simulink library "dsparch4"  (Simulink 6.0)
settings: Solver=ode45  SolverMode=SingleTasking  StartTime=0.0  StopTime=10.0  RelTol=1e-3
values from neighbouring files (symbols this model uses):
  a = []    [dspfdes.m]    (also in dsprprim.m = a-Mi)
  b = []    [dspfdes.m]    (also in dsprprim.m = b+Li)
  c = []    [dspfdes.m]    (also in liblinks.m = cell2struct(v,f,1); sbufscop.m = 'auto')
  d = []    [dspfdes.m]    (also in dsprprim.m = ['x[' num2str(Mi) 'n/' num2str(Li) ']']; resave_mdl.m = dir('*.mdl'); sbufscop.m = abs(magMax-magMin); sdspfscope.m = get(block_data.hframenum(2),'userdata'))
  H = reshape(H,Li,Mi*Ni)    [dsprprim.m]
  N = size(cmap,1)    [sdspmview.m]
undefined symbols (not defined in the file or in its folder): bitrevorder, D, dspblkfdatool, L, M
libraries: dspmtrx3 x7, dspsigattribs x4, dspxfrm3 x4, dspbuff3 x4, dspsigops x2, dsparch4 x1, simulink x1
settings Model: Creator=hshivaku  LastModifiedBy=hshivaku  ExtModeAutoUpdateStatusClock=off  ProdHWDeviceType=Specified
settings DataIOCC: SignalLoggingName=logsOut
settings OptimizationCC: BooleanDataType=off
settings DebuggingCC: CheckExecutionContextPreStartOutputMsg=on  CheckExecutionContextRuntimeOutputMsg=on  SolverPrmCheckMsg=none
settings HardwareCC: ProdHWDeviceType=Specified  TargetUnknown=on
settings ModelReferenceCC: UpdateModelReferenceTargets=IfOutOfDate
settings SFSimCC: SFSimApplyToAllLibs=on  SFSimBuildMode=Incremental

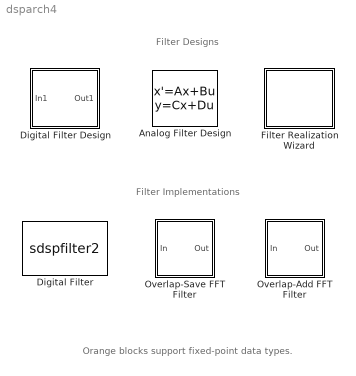
== system dsparch4 ==
  note: Filter Designs
  note: Filter Implementations
  note: Orange blocks support fixed-point data types.
  Analog Filter Design : StateSpace  A=a  B=b  C=c  D=d  mask(Analog Filter Design){method=Butterworth, filttype=Lowpass, N=8, Wlo=30, Whi=80, Rp=2, Rs=40}
      mask prompts: method "Design method:"; filttype "Filter type:"; N "Filter order:"; Wlo "Passband edge frequency (rads/sec):"; Whi "(unused)"; Rp "Passband ripple in dB:"; Rs "Stopband attenuation in dB:"
      mask help: Design one of several standard analog filters, implemented in state-space form.
      mask init:
      | [a,b,c,d,h,w,str]=dspblkanalog('design', method,filttype,N,Wlo,Whi,Rp,Rs);
      mask Help: web(dspbhelp);
      mask StyleString: popup(Butterworth|Chebyshev I|Chebyshev II|Elliptic|Bessel),popup(Lowpass|Highpass|Bandpass|Bandstop),edit,edit,edit,edit,edit
      mask CallbackString: dspblkanalog|dspblkanalog|||||
      mask Display: plot(w,h); text(.05,.9,str);
  Digital Filter Design : Subsystem  StartFcn=dspblkfdatool('StartFcn');  TreatAsAtomicUnit=on  PropExecContextAcrossSSBoundary=on
      mask init:
      | h = dspblkfdatool('initializationCommands');
      settings: ModelCloseFcn=dspblkfdatool('ModelCloseFcn');  NameChangeFcn=dspblkfdatool('NameChange');  OpenFcn=dspblkfdatool('OpenFcn');  CloseFcn=dspblkfdatool('CloseFcn');
      mask Display:
      | plot(h);
      | text(.05,.9,'FDATool')
  Digital Filter : S-Function  DialogController=dspDDGCreate  DialogControllerArgs=DataTag2  FunctionName=sdspfilter2  Parameters=a.CoeffsFromMask, a.FilterType, a.FilterStruct, a.FilterPerSample, a.a0CoeffIsUnity, a.Coeff1, a.Coeff2, a.sosCoeffs, a.scaleValues, a.IC, secondCoeffFracLength, scaleValueFracLength, tapSumMode, tapSumWordLength, tapSumFracLength, stageIOMode, stageIOWordLength, stageInFracLength, stageOutFracLength, dtInfo.firstCoeffMode, dtInfo.firstCoeffWordLength, dtInfo.firstCoeffFracLength, dtInfo.prodOutputMode, dtInfo.prodOutputWordLength, dtInfo.prodOutputFracLength, dtInfo.accumMode, dtInfo.accumWordLength, dtInfo.accumFracLength, dtInfo.memoryMode, dtInfo.memoryWordLength, dtInfo.memoryFracLength, dtInfo.outputMode, dtInfo.outputWordLength, dtInfo.outputFracLength, dtInfo.roundingMode, dtInfo.overflowMode  mask(Digital Filter){TypePopup=IIR (poles & zeros), IIRFiltStruct=Direct form II transposed, AllPoleFiltStruct=Direct form, FIRFiltStruct=Direct form, CoeffSource=Specify via dialog, NumCoeffs=[1 2], DenCoeffs=[1 0.1], BiQuadCoeffs=[1 0.3 0.4 1 0.1 0.2], LatticeCoeffs=[0.2 0.4], denIgnore=on, FiltPerSampPopup=One filter per frame, IC=0, ICnum=0, ICden=0, additionalParams=off, allowOverrides=on, showCoeff=off, firstCoeffMode=Same word length as input, firstCoeffWordLength=16, firstCoeffFracLength=15, secondCoeffMode=Same as numerator, secondCoeffWordLength=16, secondCoeffFracLength=15, thirdCoeffMode=Same as input, thirdCoeffWordLength=16, thirdCoeffFracLength=15, showOut=off, outputMode=Same as accumulator, outputWordLength=16, outputFracLength=15, showAcc=off, accumMode=Same as product output, accumWordLength=32, accumFracLength=30, showMpy=off, prodOutputMode=Same as input, prodOutputWordLength=32, prodOutputFracLength=30, showMem=off, memoryMode=Same as accumulator, memoryWordLength=16, memoryFracLength=15, roundingMode=Floor, overflowMode=off, ScaleValues=1, scaleValueFracLength=14, tapSumMode=Same as input, tapSumWordLength=32, tapSumFracLength=30, stageIOMode=Same as input, stageIOWordLength=16, stageInFracLength=15, stageOutFracLength=15, LockScale=off}
      mask prompts: TypePopup "Transfer function type:"; IIRFiltStruct "Filter structure:"; AllPoleFiltStruct "Filter structure:"; FIRFiltStruct "Filter structure:"; CoeffSource "Coefficient source:"; NumCoeffs "Numerator coefficients:"; DenCoeffs "Denominator coefficients:"; BiQuadCoeffs "SOS matrix (Mx6):"; LatticeCoeffs "Reflection coefficients:"; denIgnore "First denominator coefficient = 1, remove 1/a0 term in the structure"; FiltPerSampPopup "Coefficient update rate:"; IC "Initial conditions:"; ICnum "Initial conditions on zeros side:"; ICden "Initial conditions on poles side:"; additionalParams "------- Show additional parameters --------"; allowOverrides "Allow overrides from DSP Fixed-Point Attributes blocks"; showCoeff "------- Show coefficient fixed-point attributes --------"; firstCoeffMode "Numerator coefficient attributes:"; firstCoeffWordLength "Numerator coefficient word length:"; firstCoeffFracLength "Numerator coefficient fraction length:"; secondCoeffMode "Denominator coefficient attributes:"; secondCoeffWordLength "Denominator coefficient word length:"; secondCoeffFracLength "Denominator coefficient fraction length:"; thirdCoeffMode "Denominator coefficient attributes:"; thirdCoeffWordLength "Denominator coefficient word length:"; thirdCoeffFracLength "Denominator coefficient fraction length:"; showOut "------- Show output fixed-point attributes --------"; outputMode "Output attributes:"; outputWordLength "Output word length:"; outputFracLength "Output fraction length:"; showAcc "------- Show accumulator fixed-point attributes --------"; accumMode "Accumulator attributes:"; accumWordLength "Accumulator word length:"; accumFracLength "Accumulator fraction length:"; showMpy "------- Show product output fixed-point attributes --------"; prodOutputMode "Product output attributes:"; prodOutputWordLength "Product output word length:"; prodOutputFracLength "Product output fraction length:"; showMem "------- Show state memory fixed-point attributes --------"; memoryMode "State memory attributes:"; memoryWordLength "State memory word length:"; memoryFracLength "State memory fraction length:"; roundingMode "Round integer calculations toward:"; overflowMode "Saturate on integer overflow"; ScaleValues "Scale values:"; scaleValueFracLength "Scale value fraction length:"; tapSumMode "Tap sum attributes:"; tapSumWordLength "Tap sum word length:"; tapSumFracLength "Tap sum fraction length:"; stageIOMode "Stage IO attributes:"; stageIOWordLength "Stage IO word length:"; stageInFracLength "Stage input fraction length:"; stageOutFracLength "Stage output fraction length:"; LockScale "Lock scaling"
      mask help:
      | Independently filter each channel of the input over time using a specified digital filter implementation.  Filter coefficients can be specified using either tunable mask dialog parameters or separate input ports (useful for time-varying coefficients).
      |
      | Time-varying coefficients are supported at one of two possible rates of coefficient update in frame-based processing.  The coefficients can update at a rate of one filter per frame (i.e. they stay constant for the duration of an input frame and change for the next frame).  Or, the coefficients can update at a rate of one filter per sample (i.e. they change with every sample in the input frame).
      mask init:
      | s           = dspblkfilter('icon');
      | [a, dtInfo] = dspblkfilter('init');
      settings: CopyFcn=dspfixptcopycallback
      mask Help: web(dspbhelp);
      mask StyleString: popup(IIR (poles & zeros)|IIR (all poles)|FIR (all zeros)),popup(Direct form I|Direct form I transposed|Direct form II|Direct form II transposed|Biquad direct form I (SOS)|Biquad direct form I transposed (SOS)|Biquad direct form II (SOS)|Biquad direct form II transposed (SOS)),popup(Direct form|Direct form transposed|Lattice AR),popup(Direct form|Direct form symmetric|Direct form antisymmetric|Direct form transposed|Lattice MA),popup(Specify via dialog|Input port(s)),edit,edit,edit,edit,checkbox,popup(One filter per frame|One filter per sample),edit,edit,edit,checkbox,checkbox,checkbox,popup(Same word length as input|Specify word length|Binary point scaling|Slope and bias scaling|Same as input|User-defined),edit,edit,popup(Same as numerator|Same word length as numerator|Same word length as input|Binary point scaling|Slope and bias scaling|Same as input|User-defined),edit,edit,popup(Same word length as input|Binary point scaling|Slope and bias scaling|Same as input|User-defined),edit,edit,checkbox,popup(Same as input|Same as accumulator|Binary point scaling|Slope and bias scaling|User-defined),edit,edit,checkbox,popup(Same as input|Same as product output|Binary point scaling|Slope and bias scaling|User-defined),edit,edit,checkbox,popup(Same as input|Binary point scaling|Slope and bias scaling|User-defined),edit,edit,checkbox,popup(Same as input|Same as accumulator|Binary point scaling|Slope and bias scaling|User-defined),edit,edit,popup(Floor|Nearest),checkbox,edit,edit,popup(Same as input|Binary point scaling|Slope and bias scaling),edit,edit,popup(Same as input|Binary point scaling|Slope and bias scaling),edit,edit,edit,checkbox
      mask Display:
      | text(0.5,0.85,s.icon,'horiz','center');
      | plot(s.x, s.y);
      | port_label('input',s.i1,s.s1);
      | port_label('input',s.i2,s.s2);
      | port_label('input',1,s.in);
      | port_label('output',1,s.out);
  Filter Realization Wizard : Subsystem  PropExecContextAcrossSSBoundary=on  mask(Filter Realization Wizard){}
      mask help: Automatically construct filter realizations with specific architectures, using sum, gain, and delay blocks.
      mask init:
      | xw=[NaN 0.8 0.8 NaN 0.687 0.743 NaN 0.64 0.72 NaN 0.710 0.743 NaN 0.8 0.8 NaN 0.913 0.857 NaN 0.96 0.88 NaN 0.808 0.792 0.961 0.978 0.808 NaN 0.825 0.808 NaN 0.961 0.944];
      | yw=[NaN 0.64 0.72 NaN 0.687 0.743 NaN 0.8 0.8 NaN 0.890 0.857 NaN 0.96 0.88 NaN 0.913 0.857 NaN 0.8 0.8 NaN 0.808 0.792 0.622 0.639 0.808 NaN 0.792 0.775 NaN 0.656 0.639];
      | 
      | xl = [.1 .7 NaN .3 .3 NaN .7 .7 NaN .3 .3 NaN .7 .7 NaN .3 .9];
      | yl = [.8 .8 NaN .8 .6 NaN .8 .6 NaN .4 .2 NaN .4 .13 NaN .2 .2];
      | xz = [.46 .54 .46 NaN .54 .59 .54 .59 NaN .61 .64 NaN .67 .67];
      | yz = [.84 .8  .76 NaN .92 .92 .86 .86 NaN .93 .93 NaN .97 .89];
      | xg = [.21 .39 .3 .21 NaN .61 .79 .7 .61];
      | yg = [.6  .6  .4 .6  NaN .6  .6  .4 .6];
      | t=(0:12)/12*2*pi;
      | xs = .07*cos(t)+.7;
      | ys = .07*sin(t)+.2;
      settings: CopyFcn=dspfixptcopycallback  OpenFcn=dspfwiz
      mask Help: web(dspbhelp);
      mask Display:
      | text(.05, .9, 'FDATool');
      | plot([[xl NaN xz NaN xg NaN xs NaN]*.9-.075 xw],
      | [[yl NaN yz NaN yg NaN ys NaN]*.9-.1 yw]);
  Overlap-Add FFT Filter : Subsystem  PropExecContextAcrossSSBoundary=on  mask(Overlap-Add FFT Filter){Nfft=64, h=fir1(20,0.2), output_complexity=Real}
      mask prompts: Nfft "FFT size:"; h "FIR coefficients:"; output_complexity "Output:"
      mask help:
      | FFT based filtering using the overlap-add algorithm. Set 'Output' to 'Complex' if either the input signal or the filter coefficients are complex.
      |
      | 'FFT Size' must equal or exceed the number of filter coefficients.  Smaller FFT sizes lead to less latency but also less computational efficiency, decreasing the benefits of frequency domain processing.
      mask init:
      | [N,H,M,L] = dspblkolapfilt('init',double(Nfft),h);
      mask Help: web(dspbhelp);
      mask StyleString: edit,edit,popup(Real|Complex)
      mask Display:
      | disp('Overlap\nAdd');
      | ... plot(log10(abs(H(1:(N/2)))))
  Overlap-Save FFT Filter : Subsystem  PropExecContextAcrossSSBoundary=on  mask(Overlap-Save FFT Filter){nfft_in=64, h=fir1(20,0.2), output_complexity=Real}
      mask prompts: nfft_in "FFT size:"; h "FIR coefficients:"; output_complexity "Output:"
      mask help:
      | FFT based filtering using the overlap-save algorithm.  Set 'Output' to 'Complex' if either the input signal or the filter coefficients are complex.
      |
      | 'FFT Size' must equal or exceed the number of filter coefficients.  Smaller FFT sizes lead to less latency but also less computational efficiency, decreasing the benefits of frequency domain processing.
      mask init:
      | [N,H,M] = dspblkolapfilt('init',double(nfft_in),h);
      mask Help: web(dspbhelp);
      mask StyleString: edit,edit,popup(Real|Complex)
      mask Display:
      | disp('Overlap\nSave');
      | ... plot(log10(abs(H(1:(nfft/2)))))

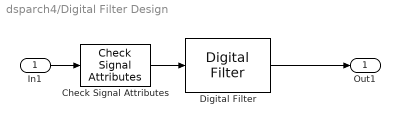
== system dsparch4/Digital Filter Design ==
  In1 : Inport  LatchInput=off
  Check Signal Attributes : dspsigattribs/Check Signal Attributes  SigAttribCheckMethod=Does not match attributes exactly  Complexity=Ignore  Frame=Ignore  DimsCheckMethod=Ignore  Dimensions=1-D  DatatypeCheckMethod=Is...  DatatypeGeneral=Floating-point  DtypeFloatSpecific=Any floating-point  DtypeFixedSpecific=Any fixed-point  DtypeIntSpecific=Any integer  SampleMode=Ignore
  Digital Filter : dsparch4/Digital Filter  DialogController=dspDDGCreate  DialogControllerArgs=DataTag1  TypePopup=FIR (all zeros)  IIRFiltStruct=Direct form II transposed  AllPoleFiltStruct=Direct form  FIRFiltStruct=Direct form  CoeffSource=Specify via dialog  NumCoeffs=[-0.00210513308421233 -0.0108086929126824 -0.0274040066202062 -0.0409457925088376 -0.0265637803556961 0.0373657306444183 0.143461670470426 0.246522720033777 0.289577286549258 0.246522720033777 0.143461670470426 0.0373657306444183 -0.0265637803556961 -0.0409457925088376 -0.0274040066202062 -0.0108086929126824 -0.00210513308421233]  DenCoeffs=[1 0.1]  BiQuadCoeffs=[1 0.3 0.4 1 0.1 0.2]  LatticeCoeffs=[0.2 0.4]  denIgnore=on  FiltPerSampPopup=One filter per frame  IC=0  ICnum=0  ICden=0  roundingMode=Floor  overflowMode=off  ScaleValues=1  scaleValueFracLength=14  stageInFracLength=15  stageOutFracLength=15
  Out1 : Outport
  wires:
  In1/1 -> Check Signal Attributes/1
  Digital Filter/1 -> Out1/1
  Check Signal Attributes/1 -> Digital Filter/1

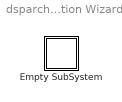
== system dsparch4/Filter Realization Wizard ==
  Empty SubSystem : Subsystem  PropExecContextAcrossSSBoundary=on

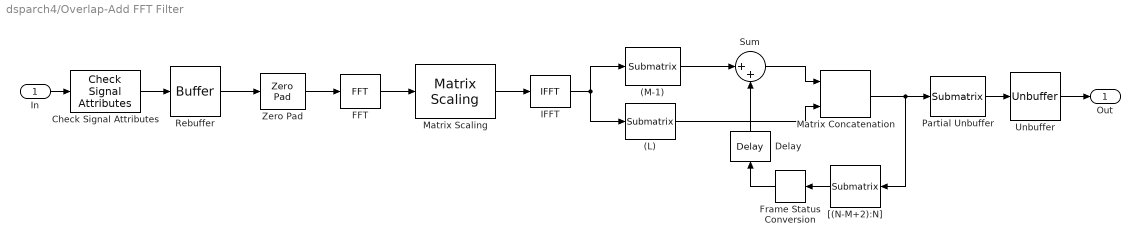
== system dsparch4/Overlap-Add FFT Filter ==
  In : Inport  LatchInput=off
  (L) : dspmtrx3/Submatrix  RowSpan=Range of rows  RowStartMode=Offset from last  RowStartIndex=L-1  RowEndMode=Last  RowEndIndex=1  ColSpan=All columns  ColStartMode=First  ColStartIndex=1  ColEndMode=Last  ColEndIndex=1
  (M-1) : dspmtrx3/Submatrix  RowSpan=Range of rows  RowStartMode=First  RowStartIndex=M-1  RowEndMode=Index  RowEndIndex=M-1  ColSpan=All columns  ColStartMode=First  ColStartIndex=1  ColEndMode=Last  ColEndIndex=1
  Check Signal Attributes : dspsigattribs/Check Signal Attributes  SigAttribCheckMethod=Does not match attributes exactly  Complexity=Ignore  Frame=Ignore  DimsCheckMethod=Ignore  Dimensions=1-D  DatatypeCheckMethod=Is...  DatatypeGeneral=Floating-point  DtypeFloatSpecific=Any floating-point  DtypeFixedSpecific=Any fixed-point  DtypeIntSpecific=Any integer  SampleMode=Ignore
  Delay : dspsigops/Delay  Orientation=up  dly_unit=Samples  delay=1  ic_detail=off  dif_ic_for_ch=off  dif_ic_for_dly=off  ic=0  reset_popup=None
  FFT : dspxfrm3/FFT  CompMethod=Table lookup  TableOpt=Speed  BitRevOrder=on  SkipNorm=on  roundingMode=Floor  overflowMode=off
      settings: allowOverrides=off
  Frame Status Conversion : dspsigattribs/Frame Status Conversion  Orientation=left  growRefPort=off  outframe=Sample-based
  IFFT : dspxfrm3/IFFT  DialogController=dspDDGCreate  DialogControllerArgs=DataTag3  CompMethod=Table lookup  TableOpt=Speed  BitRevOrder=on  cs_in=on  SkipNorm=off  mode=Real  roundingMode=Floor  overflowMode=off
      settings: allowOverrides=off
  Matrix Concatenation : simulink/Math Operations/Matrix Concatenation  numInports=2  catMethod=Vertical
  Matrix Scaling : dspmtrx3/Matrix Scaling  mode=Scale rows (D*A)  D_Source=Dialog parameter  D_VectFromMask=bitrevorder(H(:))  roundingMode=Floor  overflowMode=off
      settings: allowOverrides=off
  Partial Unbuffer : dspmtrx3/Submatrix  RowSpan=Range of rows  RowStartMode=First  RowStartIndex=M  RowEndMode=Index  RowEndIndex=L  ColSpan=All columns  ColStartMode=First  ColStartIndex=1  ColEndMode=Last  ColEndIndex=1
  Rebuffer : dspbuff3/Buffer  N=L  V=0  ic=0
  Sum : Sum  Inputs=|++  InputSameDT=on
  Unbuffer : dspbuff3/Unbuffer  ic=0
  Zero Pad : dspsigops/Zero Pad  padSigAt=End  zpadAlong=Columns  padNumOutRowsSpecMethod=User-specified  numOutRows=N  padNumOutColsSpecMethod=User-specified  numOutCols=1  trunc_flag=None
  "[(N-M+2):N]" : dspmtrx3/Submatrix  Orientation=left  RowSpan=Range of rows  RowStartMode=Index  RowStartIndex=(N-M+2)  RowEndMode=Last  RowEndIndex=N  ColSpan=All columns  ColStartMode=First  ColStartIndex=1  ColEndMode=Last  ColEndIndex=1
  Out : Outport  InitialOutput=0
  wires:
  Partial Unbuffer/1 -> Unbuffer/1
  Sum/1 -> Matrix Concatenation/1
  (M-1)/1 -> Sum/1
  Delay/1 -> Sum/2
  (L)/1 -> Matrix Concatenation/2
  "[(N-M+2):N]"/1 -> Frame Status Conversion/1
  Matrix Concatenation/1 -> Partial Unbuffer/1, "[(N-M+2):N]"/1
  Unbuffer/1 -> Out/1
  Matrix Scaling/1 -> IFFT/1
  IFFT/1 -> (L)/1, (M-1)/1
  Zero Pad/1 -> FFT/1
  Rebuffer/1 -> Zero Pad/1
  FFT/1 -> Matrix Scaling/1
  In/1 -> Check Signal Attributes/1
  Frame Status Conversion/1 -> Delay/1
  Check Signal Attributes/1 -> Rebuffer/1

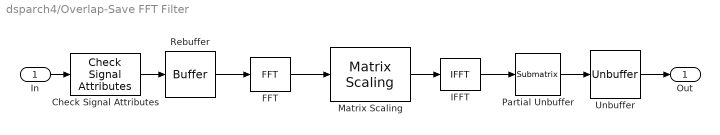
== system dsparch4/Overlap-Save FFT Filter ==
  In : Inport  LatchInput=off
  Check Signal Attributes : dspsigattribs/Check Signal Attributes  SigAttribCheckMethod=Does not match attributes exactly  Complexity=Ignore  Frame=Ignore  DimsCheckMethod=Ignore  Dimensions=1-D  DatatypeCheckMethod=Is...  DatatypeGeneral=Floating-point  DtypeFloatSpecific=Any floating-point  DtypeFixedSpecific=Any fixed-point  DtypeIntSpecific=Any integer  SampleMode=Ignore
  FFT : dspxfrm3/FFT  CompMethod=Table lookup  TableOpt=Speed  BitRevOrder=on  SkipNorm=on  roundingMode=Floor  overflowMode=off
      settings: allowOverrides=off
  IFFT : dspxfrm3/IFFT  DialogController=dspDDGCreate  DialogControllerArgs=DataTag4  CompMethod=Table lookup  TableOpt=Speed  BitRevOrder=on  cs_in=on  SkipNorm=off  mode=Real  roundingMode=Floor  overflowMode=off
      settings: allowOverrides=off
  Matrix Scaling : dspmtrx3/Matrix Scaling  mode=Scale rows (D*A)  D_Source=Dialog parameter  D_VectFromMask=bitrevorder(H(:))  roundingMode=Floor  overflowMode=off
      settings: allowOverrides=off
  Partial Unbuffer : dspmtrx3/Submatrix  RowSpan=Range of rows  RowStartMode=Index  RowStartIndex=M  RowEndMode=Last  RowEndIndex=1  ColSpan=All columns  ColStartMode=First  ColStartIndex=1  ColEndMode=Last  ColEndIndex=1
  Rebuffer : dspbuff3/Buffer  N=N  V=M-1  ic=0
  Unbuffer : dspbuff3/Unbuffer  ic=0
  Out : Outport  InitialOutput=0
  wires:
  Unbuffer/1 -> Out/1
  Partial Unbuffer/1 -> Unbuffer/1
  IFFT/1 -> Partial Unbuffer/1
  Matrix Scaling/1 -> IFFT/1
  Rebuffer/1 -> FFT/1
  FFT/1 -> Matrix Scaling/1
  In/1 -> Check Signal Attributes/1
  Check Signal Attributes/1 -> Rebuffer/1

== system dsparch4/Filter Realization Wizard/Empty SubSystem ==
